simulink model "Model_following"  (R2023a)
settings: Solver=FixedStepAuto  StartTime=0.0  StopTime=stop_time  FixedStep=sample_time  RelTol=1e-3
values from neighbouring files (symbols this model uses):
  lambda = 0.95    [example4.m]
  n_a = 2    [example4.m]
  n_b = 2    [example4.m]
  P0 = diag([100 100 1 1])    [example4.m]    (also in example7.m = 10*eye(4))
  sample_time = 0.5    [example4.m]    (also in example6.m = 0.01)
  stop_time = 150    [example4.m]    (also in example6.m = 100)
  theta0 = [0; 0; 0.01; 0.2]    [example4.m]    (also in example7.m = [1 0 0 0]')
undefined symbols (not defined in the file or in its folder): r, s
libraries: simulink x4
settings Model: Creator=Mmoha  LastModifiedBy=Mmoha

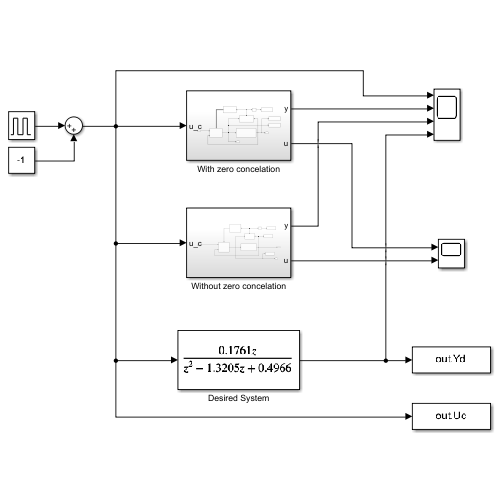
[thumbnail: Simulink's stored preview of the top-level diagram]
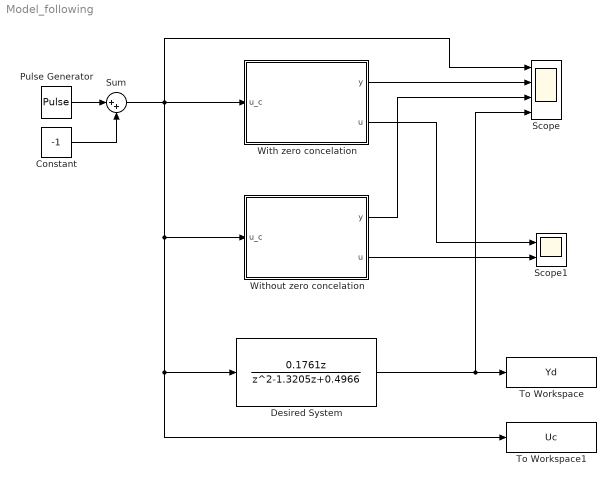
== system Model_following ==
  Constant : Constant  Value=-1
  Desired System : DiscreteTransferFcn  Numerator=[0.1761 0]  Denominator=[1 -1.3205 0.4966]  SampleTime=sample_time  a0EqualsOne=on
  Pulse Generator : DiscretePulseGenerator  PulseType=Time based  Amplitude=2  Period=50  PulseWidth=50
  Scope : Scope  NumInputPorts=4
  Scope1 : Scope  NumInputPorts=2
  Sum : Sum  Inputs=|++
  To Workspace : ToWorkspace  VariableName=Yd  SaveFormat=Timeseries  SampleTime=-1
  To Workspace1 : ToWorkspace  VariableName=Uc  SaveFormat=Timeseries  SampleTime=-1
  With zero concelation : Subsystem
  Without zero concelation : Subsystem
  wires:
  Sum/1 -> With zero concelation/1(u_c), Scope/1, To Workspace1/1, Desired System/1, Without zero concelation/1(u_c)
  Desired System/1 -> To Workspace/1, Scope/4
  With zero concelation/1(y) -> Scope/2
  With zero concelation/2(u) -> Scope1/1
  Without zero concelation/2(u) -> Scope1/2
  Without zero concelation/1(y) -> Scope/3
  Pulse Generator/1 -> Sum/1
  Constant/1 -> Sum/2

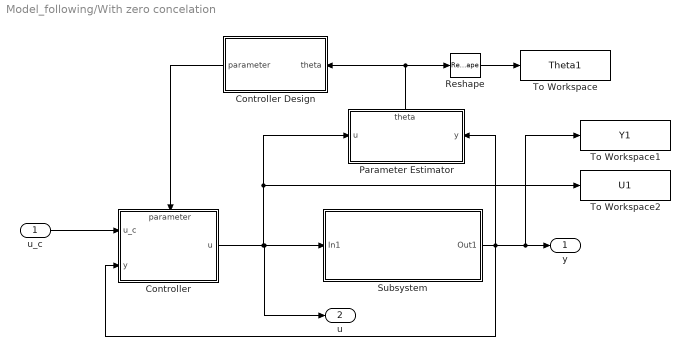
== system Model_following/With zero concelation ==
  u_c : Inport
  Controller : Subsystem
      settings: PortSchema="{\"entries\":[{\"content\":{\"sides\":[{\"content\":{\"connectorIds\":[\"In1\",\"In2\"]},\"type\":\"ConnectorPlacement.EquallySpacedRectSide\",\"uuid\":\"de166d03-2574-4be9-91e3-f68e474131a4\"},{\"content\":{\"connectorIds\":[\"Out1\"],\"side\":\"RIGHT\"},\"type\":\"ConnectorPlacement.EquallySpacedRectSide\",\"uuid\":\"3d5de88b-6c54-47ab-9bd7-fa8a92892563\"},{\"content\":{\"connectorIds\":[\"In3\"],\"side\":\"TOP\"},\"type\":\"ConnectorPlacement.EquallySpacedRectSide\",\"uuid\":\"159bb116-3d7f-46ea-9607-14d6ab0b54b0\"}]},\"type\":\"ConnectorPlacement.EquallySpacedConnector\",\"uuid\":\"b1147f71-a126-4863-a65e-99bf87cd0c97\"}],\"packageUris\":[\"http://schema.mathworks.com/mf0/Connector/R2020b\"],\"version\":\"1.0\"}"
  Controller Design : Subsystem
      settings: PortSchema="{\"entries\":[{\"content\":{\"sides\":[{\"content\":{\"connectorIds\":[\"Out1\"]},\"type\":\"ConnectorPlacement.EquallySpacedRectSide\",\"uuid\":\"53e8d639-ecea-4436-a4b4-423671f8abf5\"},{\"content\":{\"connectorIds\":[\"In1\"],\"side\":\"RIGHT\"},\"type\":\"ConnectorPlacement.EquallySpacedRectSide\",\"uuid\":\"db5d5234-b438-48d2-9c76-1224fbffd4fc\"},{\"content\":{\"side\":\"TOP\"},\"type\":\"ConnectorPlacement.EquallySpacedRectSide\",\"uuid\":\"484a8bd1-bf0a-48d9-87ad-08e804bbed03\"}]},\"type\":\"ConnectorPlacement.EquallySpacedConnector\",\"uuid\":\"1af6c988-92d8-45e5-8cd5-deae15ac0af0\"}],\"packageUris\":[\"http://schema.mathworks.com/mf0/Connector/R2020b\"],\"version\":\"1.0\"}"
  Parameter Estimator : Subsystem
      settings: PortSchema="{\"entries\":[{\"content\":{\"sides\":[{\"content\":{\"connectorIds\":[\"In1\"]},\"type\":\"ConnectorPlacement.EquallySpacedRectSide\",\"uuid\":\"de166d03-2574-4be9-91e3-f68e474131a4\"},{\"content\":{\"connectorIds\":[\"In2\"],\"side\":\"RIGHT\"},\"type\":\"ConnectorPlacement.EquallySpacedRectSide\",\"uuid\":\"3d5de88b-6c54-47ab-9bd7-fa8a92892563\"},{\"content\":{\"connectorIds\":[\"Out1\"],\"side\":\"TOP\"},\"type\":\"ConnectorPlacement.EquallySpacedRectSide\",\"uuid\":\"159bb116-3d7f-46ea-9607-14d6ab0b54b0\"}]},\"type\":\"ConnectorPlacement.EquallySpacedConnector\",\"uuid\":\"b1147f71-a126-4863-a65e-99bf87cd0c97\"}],\"packageUris\":[\"http://schema.mathworks.com/mf0/Connector/R2020b\"],\"version\":\"1.0\"}"
  Reshape : Reshape
  Subsystem : Subsystem  Variant=on  VariantControlMode=label  VariantControl=Choice  LabelModeActiveChoice=Choice_1
  To Workspace : ToWorkspace  VariableName=Theta1  SaveFormat=Timeseries  SampleTime=-1
  To Workspace1 : ToWorkspace  VariableName=Y1  SaveFormat=Timeseries  SampleTime=-1
  To Workspace2 : ToWorkspace  VariableName=U1  SaveFormat=Timeseries  SampleTime=-1
  y : Outport
  u : Outport  Port=2
  wires:
  u_c/1 -> Controller/1(u_c)
  Controller Design/1(parameter) -> Controller/3(parameter)
  Controller/1(u) -> Subsystem/1(In1), u/1, To Workspace2/1, Parameter Estimator/1(u)
  Parameter Estimator/1(theta) -> Controller Design/1(theta), Reshape/1
  Reshape/1 -> To Workspace/1
  Subsystem/1(Out1) -> Controller/2(y), y/1, To Workspace1/1, Parameter Estimator/2(y)

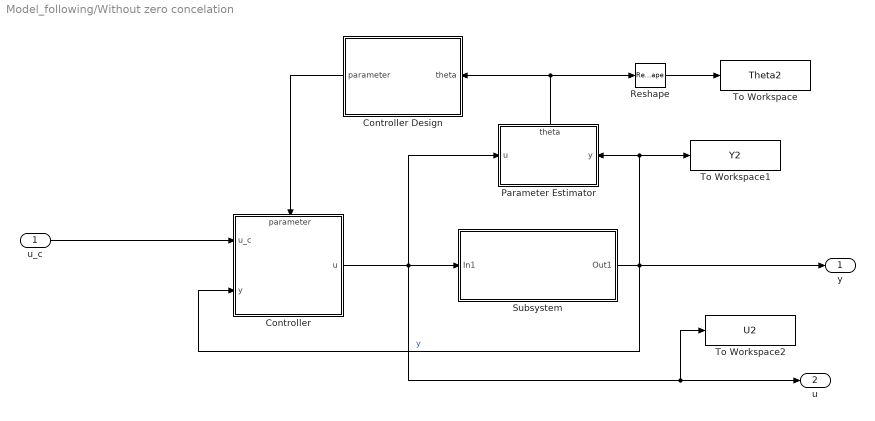
== system Model_following/Without zero concelation ==
  u_c : Inport
  Controller : Subsystem
      settings: PortSchema="{\"entries\":[{\"content\":{\"sides\":[{\"content\":{\"connectorIds\":[\"In1\",\"In2\"]},\"type\":\"ConnectorPlacement.EquallySpacedRectSide\",\"uuid\":\"de166d03-2574-4be9-91e3-f68e474131a4\"},{\"content\":{\"connectorIds\":[\"Out1\"],\"side\":\"RIGHT\"},\"type\":\"ConnectorPlacement.EquallySpacedRectSide\",\"uuid\":\"3d5de88b-6c54-47ab-9bd7-fa8a92892563\"},{\"content\":{\"connectorIds\":[\"In3\"],\"side\":\"TOP\"},\"type\":\"ConnectorPlacement.EquallySpacedRectSide\",\"uuid\":\"159bb116-3d7f-46ea-9607-14d6ab0b54b0\"}]},\"type\":\"ConnectorPlacement.EquallySpacedConnector\",\"uuid\":\"b1147f71-a126-4863-a65e-99bf87cd0c97\"}],\"packageUris\":[\"http://schema.mathworks.com/mf0/Connector/R2020b\"],\"version\":\"1.0\"}"
  Controller Design : Subsystem
      settings: PortSchema="{\"entries\":[{\"content\":{\"sides\":[{\"content\":{\"connectorIds\":[\"Out1\"]},\"type\":\"ConnectorPlacement.EquallySpacedRectSide\",\"uuid\":\"53e8d639-ecea-4436-a4b4-423671f8abf5\"},{\"content\":{\"connectorIds\":[\"In1\"],\"side\":\"RIGHT\"},\"type\":\"ConnectorPlacement.EquallySpacedRectSide\",\"uuid\":\"db5d5234-b438-48d2-9c76-1224fbffd4fc\"},{\"content\":{\"side\":\"TOP\"},\"type\":\"ConnectorPlacement.EquallySpacedRectSide\",\"uuid\":\"484a8bd1-bf0a-48d9-87ad-08e804bbed03\"}]},\"type\":\"ConnectorPlacement.EquallySpacedConnector\",\"uuid\":\"1af6c988-92d8-45e5-8cd5-deae15ac0af0\"}],\"packageUris\":[\"http://schema.mathworks.com/mf0/Connector/R2020b\"],\"version\":\"1.0\"}"
  Parameter Estimator : Subsystem
      settings: PortSchema="{\"entries\":[{\"content\":{\"sides\":[{\"content\":{\"connectorIds\":[\"In1\"]},\"type\":\"ConnectorPlacement.EquallySpacedRectSide\",\"uuid\":\"de166d03-2574-4be9-91e3-f68e474131a4\"},{\"content\":{\"connectorIds\":[\"In2\"],\"side\":\"RIGHT\"},\"type\":\"ConnectorPlacement.EquallySpacedRectSide\",\"uuid\":\"3d5de88b-6c54-47ab-9bd7-fa8a92892563\"},{\"content\":{\"connectorIds\":[\"Out1\"],\"side\":\"TOP\"},\"type\":\"ConnectorPlacement.EquallySpacedRectSide\",\"uuid\":\"159bb116-3d7f-46ea-9607-14d6ab0b54b0\"}]},\"type\":\"ConnectorPlacement.EquallySpacedConnector\",\"uuid\":\"b1147f71-a126-4863-a65e-99bf87cd0c97\"}],\"packageUris\":[\"http://schema.mathworks.com/mf0/Connector/R2020b\"],\"version\":\"1.0\"}"
  Reshape : Reshape
  Subsystem : Subsystem  Variant=on  VariantControlMode=label  VariantControl=Choice  LabelModeActiveChoice=Choice_1
  To Workspace : ToWorkspace  VariableName=Theta2  SaveFormat=Timeseries  SampleTime=-1
  To Workspace1 : ToWorkspace  VariableName=Y2  SaveFormat=Timeseries  SampleTime=-1
  To Workspace2 : ToWorkspace  VariableName=U2  SaveFormat=Timeseries  SampleTime=-1
  y : Outport
  u : Outport  Port=2
  wires:
  Parameter Estimator/1(theta) -> Reshape/1, Controller Design/1(theta)
  Controller/1(u) -> Subsystem/1(In1), Parameter Estimator/1(u), To Workspace2/1, u/1
  Subsystem/1(Out1) -> Parameter Estimator/2(y), To Workspace1/1, Controller/2(y), y/1  "y"
  Controller Design/1(parameter) -> Controller/3(parameter)
  u_c/1 -> Controller/1(u_c)
  Reshape/1 -> To Workspace/1

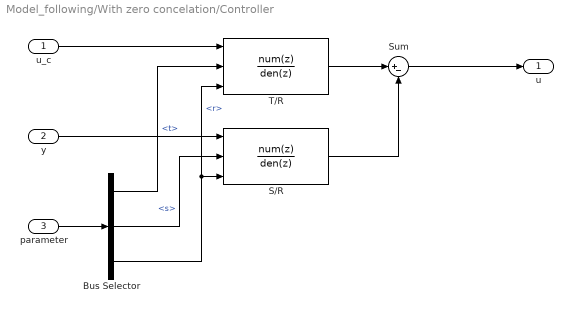
== system Model_following/With zero concelation/Controller ==
  u_c : Inport
  y : Inport  Port=2
  parameter : Inport  Port=3
  Bus Selector : BusSelector  OutputSignals=t,s,r
  S/R : DiscreteTransferFcn  NumeratorSource=Input port  DenominatorSource=Input port  SampleTime=sample_time  a0EqualsOne=on
      settings: InputPortMap=u0,p1,p3
  Sum : Sum  Inputs=|+-
  T/R : DiscreteTransferFcn  NumeratorSource=Input port  DenominatorSource=Input port  SampleTime=sample_time  a0EqualsOne=on
      settings: InputPortMap=u0,p1,p3
  u : Outport
  wires:
  y/1 -> S/R/1
  T/R/1 -> Sum/1
  parameter/1 -> Bus Selector/1
  u_c/1 -> T/R/1
  S/R/1 -> Sum/2
  Bus Selector/1 -> T/R/2  "<t>"
  Bus Selector/2 -> S/R/2  "<s>"
  Bus Selector/3 -> T/R/3, S/R/3  "<r>"
  Sum/1 -> u/1

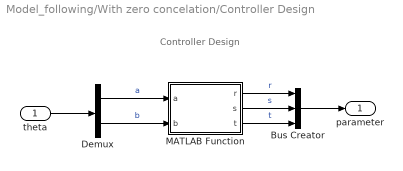
== system Model_following/With zero concelation/Controller Design ==
  note: Controller Design
  theta : Inport
  Bus Creator : BusCreator  Inputs=r,s,t
  Demux : Demux  Outputs=[n_a, n_b]
  MATLAB Function : MATLAB Function  TreatAsAtomicUnit=on
  parameter : Outport
  wires:
  Demux/1 -> MATLAB Function/1(a)  "a"
  theta/1 -> Demux/1
  Demux/2 -> MATLAB Function/2(b)  "b"
  MATLAB Function/1(r) -> Bus Creator/1  "r"
  MATLAB Function/2(s) -> Bus Creator/2  "s"
  MATLAB Function/3(t) -> Bus Creator/3  "t"
  Bus Creator/1 -> parameter/1

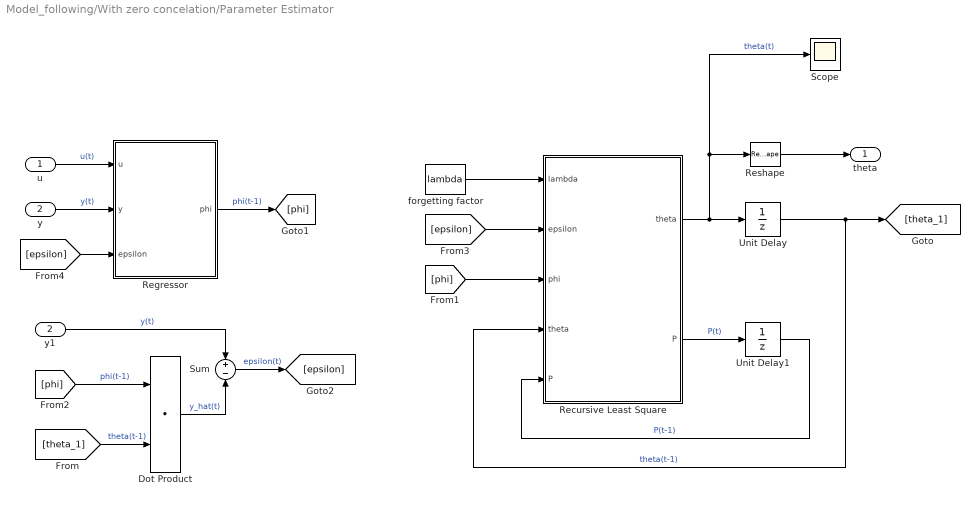
== system Model_following/With zero concelation/Parameter Estimator ==
  u : Inport
  y : Inport  Port=2
  Dot Product : DotProduct  OutDataTypeStr=Inherit: Inherit via internal rule
  Recursive Least Square : MATLAB Function  TreatAsAtomicUnit=on  VariantControl=(default)
  Regressor : Subsystem  VariantControl=(default)
  Reshape : Reshape  OutputDimensionality=Row vector (2-D)
  Scope : Scope
  Sum : Sum  Inputs=+|-
  Unit Delay : UnitDelay  InitialCondition=theta0  SampleTime=sample_time  HasFrameUpgradeWarning=on
  Unit Delay1 : UnitDelay  InitialCondition=P0  SampleTime=sample_time  HasFrameUpgradeWarning=on
  forgetting factor : Constant  Value=lambda
  y1 : InportShadow  Port=2
  theta : Outport
  wires:
  [phi] -> Recursive Least Square/3(phi)
  forgetting factor/1 -> Recursive Least Square/1(lambda)
  [epsilon] -> Recursive Least Square/2(epsilon)
  Unit Delay/1 -> [theta_1], Recursive Least Square/4("theta ")  "theta(t-1)"
  u/1 -> Regressor/1(u)  "u(t)"
  Unit Delay1/1 -> Recursive Least Square/5("P ")  "P(t-1)"
  [epsilon] -> Regressor/3(epsilon)
  Dot Product/1 -> Sum/2  "y_hat(t)"
  Regressor/1(phi) -> [phi]  "phi(t-1)"
  y/1 -> Regressor/2(y)  "y(t)"
  [phi] -> Dot Product/1  "phi(t-1)"
  [theta_1] -> Dot Product/2  "theta(t-1)"
  Recursive Least Square/1(theta) -> Scope/1, Reshape/1, Unit Delay/1  "theta(t)"
  Recursive Least Square/2(P) -> Unit Delay1/1  "P(t)"
  y1/1 -> Sum/1  "y(t)"
  Sum/1 -> [epsilon]  "epsilon(t)"
  Reshape/1 -> theta/1

== system Model_following/With zero concelation/Subsystem ==
  In1 : Inport
  TimeInvariant : Subsystem  VariantControl=Choice
  TimeVarying : Subsystem  VariantControl=Choice_1
  Out1 : Outport

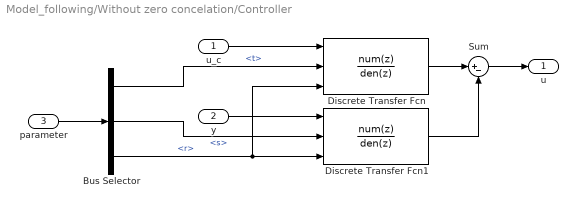
== system Model_following/Without zero concelation/Controller ==
  u_c : Inport
  y : Inport  Port=2
  parameter : Inport  Port=3
  Bus Selector : BusSelector  OutputSignals=t,s,r
  Discrete Transfer Fcn : DiscreteTransferFcn  NumeratorSource=Input port  DenominatorSource=Input port  SampleTime=sample_time  a0EqualsOne=on
      settings: InputPortMap=u0,p1,p3
  Discrete Transfer Fcn1 : DiscreteTransferFcn  NumeratorSource=Input port  DenominatorSource=Input port  SampleTime=sample_time  a0EqualsOne=on
      settings: InputPortMap=u0,p1,p3
  Sum : Sum  Inputs=|+-
  u : Outport
  wires:
  Sum/1 -> u/1
  Bus Selector/3 -> Discrete Transfer Fcn1/3, Discrete Transfer Fcn/3  "<r>"
  Bus Selector/2 -> Discrete Transfer Fcn1/2  "<s>"
  Bus Selector/1 -> Discrete Transfer Fcn/2  "<t>"
  Discrete Transfer Fcn1/1 -> Sum/2
  u_c/1 -> Discrete Transfer Fcn/1
  parameter/1 -> Bus Selector/1
  Discrete Transfer Fcn/1 -> Sum/1
  y/1 -> Discrete Transfer Fcn1/1

== system Model_following/Without zero concelation/Controller Design ==
  theta : Inport
  Bus Creator : BusCreator  Inputs=r,s,t
  Demux : Demux  Outputs=[n_a, n_b]
  MATLAB Function : MATLAB Function  TreatAsAtomicUnit=on
  parameter : Outport
  wires:
  Bus Creator/1 -> parameter/1
  MATLAB Function/3(t) -> Bus Creator/3  "t"
  MATLAB Function/2(s) -> Bus Creator/2  "s"
  MATLAB Function/1(r) -> Bus Creator/1  "r"
  Demux/2 -> MATLAB Function/2(b)  "b"
  theta/1 -> Demux/1
  Demux/1 -> MATLAB Function/1(a)  "a"

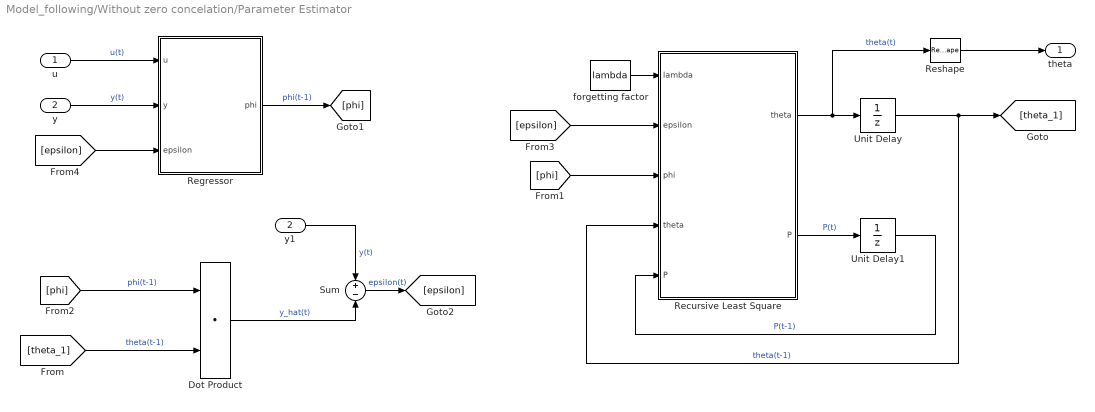
== system Model_following/Without zero concelation/Parameter Estimator ==
  u : Inport
  y : Inport  Port=2
  Dot Product : DotProduct  OutDataTypeStr=Inherit: Inherit via internal rule
  Recursive Least Square : MATLAB Function  TreatAsAtomicUnit=on  VariantControl=(default)
  Regressor : Subsystem  VariantControl=(default)
  Reshape : Reshape  OutputDimensionality=Row vector (2-D)
  Sum : Sum  Inputs=+|-
  Unit Delay : UnitDelay  InitialCondition=theta0  SampleTime=sample_time  HasFrameUpgradeWarning=on
  Unit Delay1 : UnitDelay  InitialCondition=P0  SampleTime=sample_time  HasFrameUpgradeWarning=on
  forgetting factor : Constant  Value=lambda
  y1 : InportShadow  Port=2
  theta : Outport
  wires:
  Reshape/1 -> theta/1
  Sum/1 -> [epsilon]  "epsilon(t)"
  y1/1 -> Sum/1  "y(t)"
  Recursive Least Square/2(P) -> Unit Delay1/1  "P(t)"
  Recursive Least Square/1(theta) -> Reshape/1, Unit Delay/1  "theta(t)"
  [theta_1] -> Dot Product/2  "theta(t-1)"
  [phi] -> Dot Product/1  "phi(t-1)"
  y/1 -> Regressor/2(y)  "y(t)"
  Regressor/1(phi) -> [phi]  "phi(t-1)"
  Dot Product/1 -> Sum/2  "y_hat(t)"
  [epsilon] -> Regressor/3(epsilon)
  Unit Delay1/1 -> Recursive Least Square/5("P ")  "P(t-1)"
  u/1 -> Regressor/1(u)  "u(t)"
  Unit Delay/1 -> [theta_1], Recursive Least Square/4("theta ")  "theta(t-1)"
  [epsilon] -> Recursive Least Square/2(epsilon)
  forgetting factor/1 -> Recursive Least Square/1(lambda)
  [phi] -> Recursive Least Square/3(phi)

== system Model_following/Without zero concelation/Subsystem ==
  In1 : Inport
  TimeInvariant : Subsystem  VariantControl=Choice
  TimeVarying : Subsystem  VariantControl=Choice_1
  Out1 : Outport

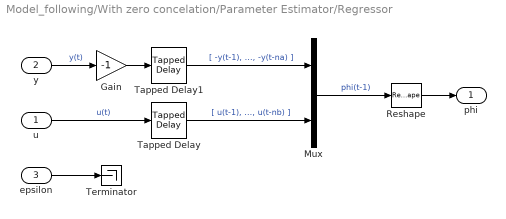
== system Model_following/With zero concelation/Parameter Estimator/Regressor ==
  u : Inport
  y : Inport  Port=2
  epsilon : Inport  Port=3
  Gain : Gain  Gain=-1
  Mux : Mux  Inputs=2
  Reshape : Reshape  OutputDimensionality=Column vector (2-D)
  Tapped Delay : simulink/Discrete/Tapped Delay  vinit=0.0  samptime=sample_time  NumDelays=n_b  DelayOrder=Newest  includeCurrent=off
  Tapped Delay1 : simulink/Discrete/Tapped Delay  vinit=0.0  samptime=sample_time  NumDelays=n_a  DelayOrder=Newest  includeCurrent=off
  Terminator : Terminator
  phi : Outport
  wires:
  Mux/1 -> Reshape/1  "phi(t-1)"
  Gain/1 -> Tapped Delay1/1
  Tapped Delay/1 -> Mux/2  "[ u(t-1), ..., u(t-nb) ]"
  Tapped Delay1/1 -> Mux/1  "[ -y(t-1), ..., -y(t-na) ]"
  y/1 -> Gain/1  "y(t)"
  u/1 -> Tapped Delay/1  "u(t)"
  Reshape/1 -> phi/1
  epsilon/1 -> Terminator/1

== system Model_following/With zero concelation/Subsystem/TimeInvariant ==
  In1 : Inport
  Discrete System : DiscreteTransferFcn  Numerator=[0 0.1065 0.0902]  Denominator=[1 -1.6065 0.6065]  SampleTime=sample_time  a0EqualsOne=on
  Out1 : Outport
  wires:
  In1/1 -> Discrete System/1
  Discrete System/1 -> Out1/1

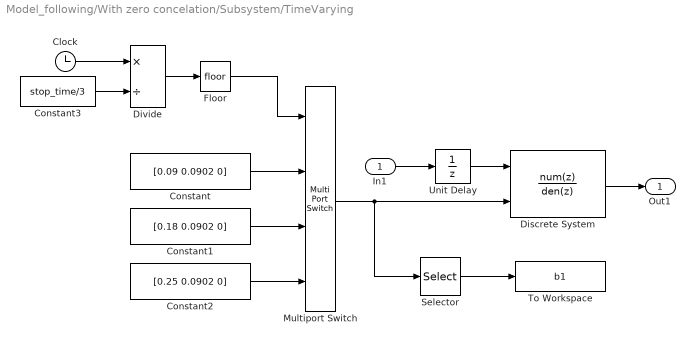
== system Model_following/With zero concelation/Subsystem/TimeVarying ==
  In1 : Inport
  Clock : Clock
  Constant : Constant  Value=[0.09 0.0902 0]
  Constant1 : Constant  Value=[0.18 0.0902 0]
  Constant2 : Constant  Value=[0.25 0.0902 0]
  Constant3 : Constant  Value=stop_time/3
  Discrete System : DiscreteTransferFcn  NumeratorSource=Input port  Numerator=[0 0.1065 0.0902]  Denominator=[1 -1.6065 0.6065]  SampleTime=sample_time  a0EqualsOne=on
      settings: InputPortMap=u0,p1
  Divide : Product  Inputs=*/
  Floor : Rounding
  Multiport Switch : MultiPortSwitch  DataPortOrder=Zero-based contiguous  DiagnosticForDefault=None  zeroidx=on  SaturateOnIntegerOverflow=off  InputSameDT=off
  Selector : Selector  InputPortWidth=3  IndexOptions=Index vector (dialog)  Indices=[1]  OutputSizes=1
  To Workspace : ToWorkspace  VariableName=b1  SaveFormat=Timeseries  SampleTime=-1
  Unit Delay : UnitDelay  SampleTime=sample_time  HasFrameUpgradeWarning=on
  Out1 : Outport
  wires:
  In1/1 -> Unit Delay/1
  Constant2/1 -> Multiport Switch/4
  Constant/1 -> Multiport Switch/2
  Constant1/1 -> Multiport Switch/3
  Clock/1 -> Divide/1
  Divide/1 -> Floor/1
  Constant3/1 -> Divide/2
  Multiport Switch/1 -> Selector/1, Discrete System/2
  Floor/1 -> Multiport Switch/1
  Discrete System/1 -> Out1/1
  Unit Delay/1 -> Discrete System/1
  Selector/1 -> To Workspace/1

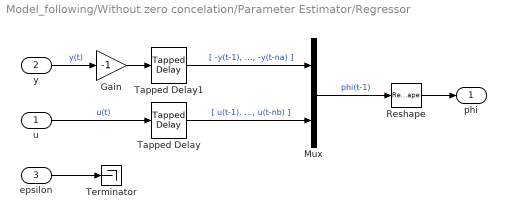
== system Model_following/Without zero concelation/Parameter Estimator/Regressor ==
  u : Inport
  y : Inport  Port=2
  epsilon : Inport  Port=3
  Gain : Gain  Gain=-1
  Mux : Mux  Inputs=2
  Reshape : Reshape  OutputDimensionality=Column vector (2-D)
  Tapped Delay : simulink/Discrete/Tapped Delay  vinit=0.0  samptime=sample_time  NumDelays=n_b  DelayOrder=Newest  includeCurrent=off
  Tapped Delay1 : simulink/Discrete/Tapped Delay  vinit=0.0  samptime=sample_time  NumDelays=n_a  DelayOrder=Newest  includeCurrent=off
  Terminator : Terminator
  phi : Outport
  wires:
  epsilon/1 -> Terminator/1
  Reshape/1 -> phi/1
  u/1 -> Tapped Delay/1  "u(t)"
  y/1 -> Gain/1  "y(t)"
  Tapped Delay1/1 -> Mux/1  "[ -y(t-1), ..., -y(t-na) ]"
  Tapped Delay/1 -> Mux/2  "[ u(t-1), ..., u(t-nb) ]"
  Gain/1 -> Tapped Delay1/1
  Mux/1 -> Reshape/1  "phi(t-1)"

== system Model_following/Without zero concelation/Subsystem/TimeInvariant ==
  In1 : Inport
  Discrete System : DiscreteTransferFcn  Numerator=[0 0.1065 0.0902]  Denominator=[1 -1.6065 0.6065]  SampleTime=sample_time  a0EqualsOne=on
  Out1 : Outport
  wires:
  In1/1 -> Discrete System/1
  Discrete System/1 -> Out1/1

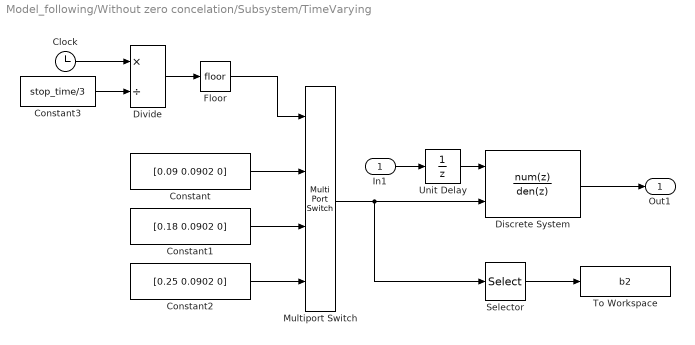
== system Model_following/Without zero concelation/Subsystem/TimeVarying ==
  In1 : Inport
  Clock : Clock
  Constant : Constant  Value=[0.09 0.0902 0]
  Constant1 : Constant  Value=[0.18 0.0902 0]
  Constant2 : Constant  Value=[0.25 0.0902 0]
  Constant3 : Constant  Value=stop_time/3
  Discrete System : DiscreteTransferFcn  NumeratorSource=Input port  Numerator=[0 0.1065 0.0902]  Denominator=[1 -1.6065 0.6065]  SampleTime=sample_time  a0EqualsOne=on
      settings: InputPortMap=u0,p1
  Divide : Product  Inputs=*/
  Floor : Rounding
  Multiport Switch : MultiPortSwitch  DataPortOrder=Zero-based contiguous  DiagnosticForDefault=None  zeroidx=on  SaturateOnIntegerOverflow=off  InputSameDT=off
  Selector : Selector  InputPortWidth=3  IndexOptions=Index vector (dialog)  Indices=[1]  OutputSizes=1
  To Workspace : ToWorkspace  VariableName=b2  SaveFormat=Timeseries  SampleTime=-1
  Unit Delay : UnitDelay  SampleTime=sample_time  HasFrameUpgradeWarning=on
  Out1 : Outport
  wires:
  In1/1 -> Unit Delay/1
  Constant2/1 -> Multiport Switch/4
  Constant/1 -> Multiport Switch/2
  Constant1/1 -> Multiport Switch/3
  Clock/1 -> Divide/1
  Divide/1 -> Floor/1
  Constant3/1 -> Divide/2
  Multiport Switch/1 -> Selector/1, Discrete System/2
  Floor/1 -> Multiport Switch/1
  Discrete System/1 -> Out1/1
  Unit Delay/1 -> Discrete System/1
  Selector/1 -> To Workspace/1

== matlab function Model_following/With zero concelation/Parameter Estimator/Recursive Least Square ==
  data: lambda input size=1; theta output; epsilon input size=1; phi input size=[n, 1]; theta input size=[n, 1]; P input size=[n, n]; P output; n parameter size=1
function [theta, P] = fcn(lambda, epsilon, phi, theta, P, n)
K = P * phi / (lambda + phi'*P*phi);
P = (eye(n) - K*phi') * P / lambda;
theta = theta + P * phi * epsilon;

== matlab function Model_following/With zero concelation/Controller Design/MATLAB Function ==
  data: r output size=[1 2]; s output size=[1 2]; a input size=[1 2]; b input size=[1 2]; t output size=[1 2]
function [r, s, t] = fcn(a, b)
am = [-1.3205, 0.4966];
bm = [0.1761, 0];
s = (am - a)/b(1);
r = [1, b(2)/b(1)];
t = [bm(1)/b(1), 0];

== matlab function Model_following/Without zero concelation/Controller Design/MATLAB Function ==
  data: r output size=[1 2]; s output size=[1 2]; a input size=[1 2]; b input size=[1 2]; t output size=[1 2]
function [r, s, t] = fcn(a, b)
am = [-1.3205, 0.4966];
a0 = 0;
Phi = [
    1,    b(1), 0;
    a(1), b(2), b(1);
    a(2), 0,    b(2)
    ];
y = [a0+am(1)-a(1); am(1)*a0+am(2)-a(2); a0*am(2)];
theta = pinv(Phi)*y;
r = [1, theta(1)];
s = [theta(2), theta(3)];
beta = (1 + am(1) + am(2)) / (b(1)+b(2));
t = [beta beta*a0];

== matlab function Model_following/Without zero concelation/Parameter Estimator/Recursive Least Square ==
  data: lambda input size=1; theta output; epsilon input size=1; phi input size=[n, 1]; theta input size=[n, 1]; P input size=[n, n]; P output; n parameter size=1
function [theta, P] = fcn(lambda, epsilon, phi, theta, P, n)
K = P * phi / (lambda + phi'*P*phi);
P = (eye(n) - K*phi') * P / lambda;
theta = theta + P * phi * epsilon;
